simulink library "DipoleField"  (R2014b)
settings: Solver=ode45  StartTime=0.0  StopTime=10.0  RelTol=1e-3
undefined symbols (not defined in the file): ConfParam
settings Model: Creator=Hp  LastModifiedBy=Hp

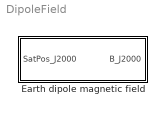
== system DipoleField ==
  Earth dipole magnetic field : Subsystem

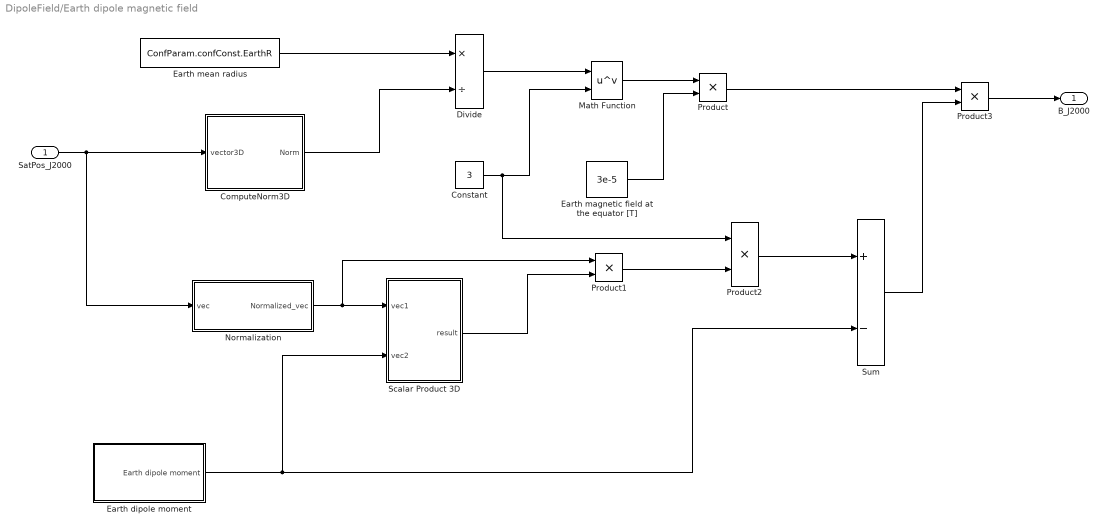
== system DipoleField/Earth dipole magnetic field ==
  SatPos_J2000 : Inport
  ComputeNorm3D : Subsystem
  Constant : Constant  Value=3
  Divide : Product  Inputs=*/
  Earth dipole moment : Subsystem
  Earth magnetic field at the equator [T] : Constant  Value=3e-5
  Earth mean radius : Constant  Value=ConfParam.confConst.EarthR
  Math Function : Math  Operator=pow  SaturateOnIntegerOverflow=on
  Normalization : Subsystem
  Product{,1..3} (4 alike) : Product
  Scalar Product 3D : Subsystem
  Sum : Sum  Inputs=+-
  B_J2000 : Outport
  wires:
  Product/1 -> Product3/1
  Product3/1 -> B_J2000/1
  Product2/1 -> Sum/1
  Math Function/1 -> Product/1
  Sum/1 -> Product3/2
  ComputeNorm3D/1(Norm) -> Divide/2
  Scalar Product 3D/1(result) -> Product1/2
  Constant/1 -> Product2/1, Math Function/2
  Product1/1 -> Product2/2
  Earth dipole moment/1(Earth dipole moment) -> Sum/2, Scalar Product 3D/2(vec2)
  SatPos_J2000/1 -> Normalization/1(vec), ComputeNorm3D/1(vector3D)
  Divide/1 -> Math Function/1
  Earth magnetic field at the equator [T]/1 -> Product/2
  Normalization/1(Normalized_vec) -> Product1/1, Scalar Product 3D/1(vec1)
  Earth mean radius/1 -> Divide/1

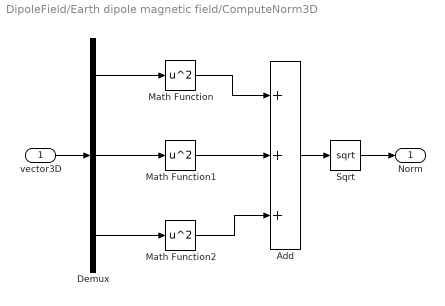
== system DipoleField/Earth dipole magnetic field/ComputeNorm3D ==
  vector3D : Inport
  Add : Sum  Inputs=+++
  Demux : Demux  Outputs=3
  Math Function : Math  Operator=square  SaturateOnIntegerOverflow=on
  Math Function1 : Math  Operator=square  SaturateOnIntegerOverflow=on
  Math Function2 : Math  Operator=square  SaturateOnIntegerOverflow=on
  Sqrt : Sqrt  SaturateOnIntegerOverflow=on
  Norm : Outport
  wires:
  vector3D/1 -> Demux/1
  Sqrt/1 -> Norm/1
  Add/1 -> Sqrt/1
  Math Function1/1 -> Add/2
  Math Function2/1 -> Add/3
  Demux/1 -> Math Function/1
  Math Function/1 -> Add/1
  Demux/3 -> Math Function2/1
  Demux/2 -> Math Function1/1

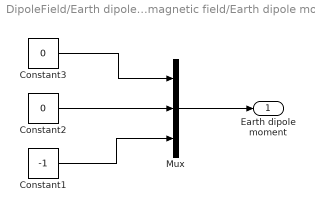
== system DipoleField/Earth dipole magnetic field/Earth dipole moment ==
  Constant1 : Constant  Value=-1
  Constant2 : Constant  Value=0
  Constant3 : Constant  Value=0
  Mux : Mux  Inputs=3
  Earth dipole moment : Outport
  wires:
  Mux/1 -> Earth dipole moment/1
  Constant2/1 -> Mux/2
  Constant3/1 -> Mux/1
  Constant1/1 -> Mux/3

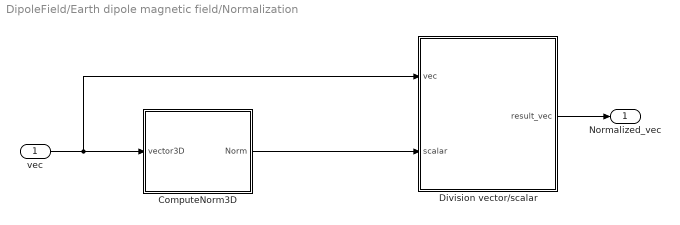
== system DipoleField/Earth dipole magnetic field/Normalization ==
  vec : Inport
  ComputeNorm3D : Subsystem
  Division vector/scalar : Subsystem
  Normalized_vec : Outport
  wires:
  ComputeNorm3D/1(Norm) -> Division vector/scalar/2(scalar)
  Division vector/scalar/1(result_vec) -> Normalized_vec/1
  vec/1 -> ComputeNorm3D/1(vector3D), Division vector/scalar/1(vec)

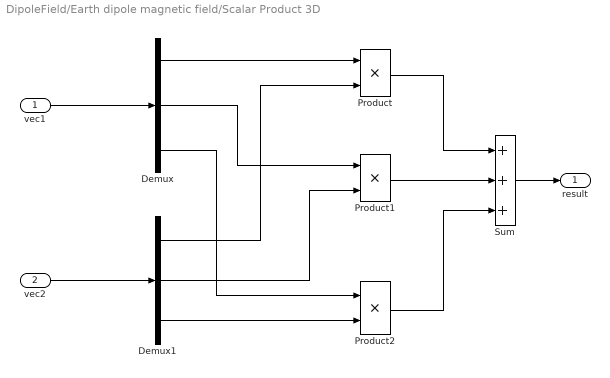
== system DipoleField/Earth dipole magnetic field/Scalar Product 3D ==
  vec1 : Inport
  vec2 : Inport  Port=2
  Demux : Demux  Outputs=3
  Demux1 : Demux  Outputs=3
  Product : Product
  Product1 : Product
  Product2 : Product
  Sum : Sum  Inputs=+++
  result : Outport
  wires:
  Product/1 -> Sum/1
  Demux/3 -> Product2/1
  Demux1/3 -> Product2/2
  Demux1/1 -> Product/2
  vec2/1 -> Demux1/1
  Product2/1 -> Sum/3
  Sum/1 -> result/1
  Demux/1 -> Product/1
  Demux/2 -> Product1/1
  Product1/1 -> Sum/2
  Demux1/2 -> Product1/2
  vec1/1 -> Demux/1

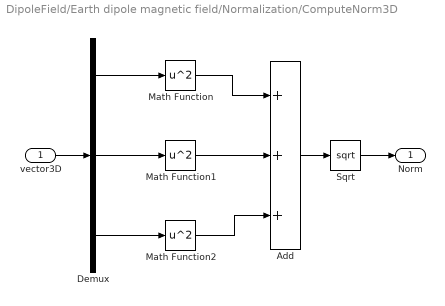
== system DipoleField/Earth dipole magnetic field/Normalization/ComputeNorm3D ==
  vector3D : Inport
  Add : Sum  Inputs=+++
  Demux : Demux  Outputs=3
  Math Function : Math  Operator=square  SaturateOnIntegerOverflow=on
  Math Function1 : Math  Operator=square  SaturateOnIntegerOverflow=on
  Math Function2 : Math  Operator=square  SaturateOnIntegerOverflow=on
  Sqrt : Sqrt  SaturateOnIntegerOverflow=on
  Norm : Outport
  wires:
  Demux/2 -> Math Function1/1
  Demux/3 -> Math Function2/1
  Math Function/1 -> Add/1
  Demux/1 -> Math Function/1
  Math Function2/1 -> Add/3
  Math Function1/1 -> Add/2
  Add/1 -> Sqrt/1
  Sqrt/1 -> Norm/1
  vector3D/1 -> Demux/1

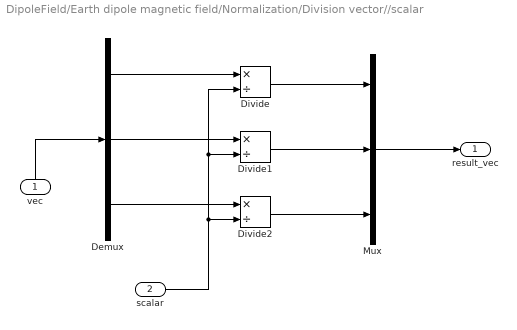
== system DipoleField/Earth dipole magnetic field/Normalization/Division vector//scalar ==
  vec : Inport
  scalar : Inport  Port=2
  Demux : Demux  Outputs=3
  Divide : Product  Inputs=*/
  Divide1 : Product  Inputs=*/
  Divide2 : Product  Inputs=*/
  Mux : Mux  Inputs=3
  result_vec : Outport
  wires:
  vec/1 -> Demux/1
  Demux/2 -> Divide1/1
  Demux/1 -> Divide/1
  Divide1/1 -> Mux/2
  Divide2/1 -> Mux/3
  Demux/3 -> Divide2/1
  scalar/1 -> Divide2/2, Divide/2, Divide1/2
  Mux/1 -> result_vec/1
  Divide/1 -> Mux/1
